simulink model "mCSControls_DG"  (R2012b)
settings: Solver=FixedStepDiscrete  StartTime=0.0  StopTime=10.0  RelTol=1e-3
values from neighbouring files (symbols this model uses):
  CDF2FThreshold = 45    [ControlCal_DG.m]
  CDF2TempThreshold = 20    [ControlCal_DG.m]
  delay = 5    [ControlCal_DG.m]
  DFThresh = 33    [ControlCal_DG.m]
  H = [90 90 90 90]    [ControlCal_DG.m]
  HeatTempThresh1 = 40    [ControlCal_DG.m]
  HeatTempThresh2 = 30    [ControlCal_DG.m]
  HeatTempThresh3 = 20    [ControlCal_DG.m]
  HStabilizationTime = 2*60    (= 120)    [ControlCal_DG.m]
  I_FAN = -1    [ControlCal_DG.m]
  I_VALVE = -1    [ControlCal_DG.m]
  initialSet = [1 1 1]    [ControlCal_DG.m]
  PBFTempThreshold = 30    [ControlCal_DG.m]
  PowerModeSwitchDelay = 30    [ControlCal_DG.m]
  SVocThresh = 550    [ControlCal_DG.m]
  T = [0 4 7 10]    [ControlCal_DG.m]
  Ts = 0.5    [ControlCal_DG.m]
  TSTempSetPoint = -2    [ControlCal_DG.m]
  TV1FThresh = 45    [ControlCal_DG.m]
  TV2FThresh = 60    [ControlCal_DG.m]
  VbatThresh = 22    [ControlCal_DG.m]
  VocDecRate = 0.5    [ControlCal_DG.m]
  VocIncrement = 5    [ControlCal_DG.m]
libraries: c2833xlib x29, simulink x23, c280xlib x11, idelinklib_tgtpref x1
(part 2 of 4)

== system mCSControls_DG/Inputs/EEPROM/EEPROMRead/AddressWrite ==
  Trigger : TriggerPort  PortDimensions=1
  Data Type Conversion : DataTypeConversion  OutDataTypeStr=uint8  RndMeth=Simplest
  I2C Transmit : c280xlib/I2C Transmit  addrFormat=7-Bit addressing  saSource=Specify via dialog  SAR=80  bitCount=8  STP=on  RM=off  STR=off
  WordAddress : Constant  Value=0  SampleTime=-1
  wires:
  WordAddress/1 -> Data Type Conversion/1
  Data Type Conversion/1 -> I2C Transmit/1

== system mCSControls_DG/Inputs/EEPROM/EEPROMRead/Receive ==
  Trigger : TriggerPort  TriggerType=falling  PortDimensions=1
  I2C Receive : c280xlib/I2C Receive  addrFormat=7-Bit addressing  saSource=Specify via dialog  SAR=80  bitCount=8  dataLength=3  initValue=initialSet  NACK=off  STP=on  STR=off  sampleTime=-1  dataType=uint8
  RD : Outport
  wires:
  I2C Receive/1 -> RD/1

== matlab function mCSControls_DG/Inputs/HMI/Data Detection ==
  data: u input; B output; M1 output; P1 output; Bp input; M1p input; P1p input
function [B,M1,P1] = fcn(u,Bp,M1p,P1p)
%#codegen

% When data length is 5 and format is [250 B M1 P 250]

n=5;
B=Bp;
M1=M1p;
P1=P1p;
for i=0:n-1
    if (u(i+1)==250 && u(mod(i+4,5)+1)==250)
        B  = u(mod(i+1,5)+1);
        M1 = u(mod(i+2,5)+1);
        P1 = u(mod(i+3,5)+1);
    end
end

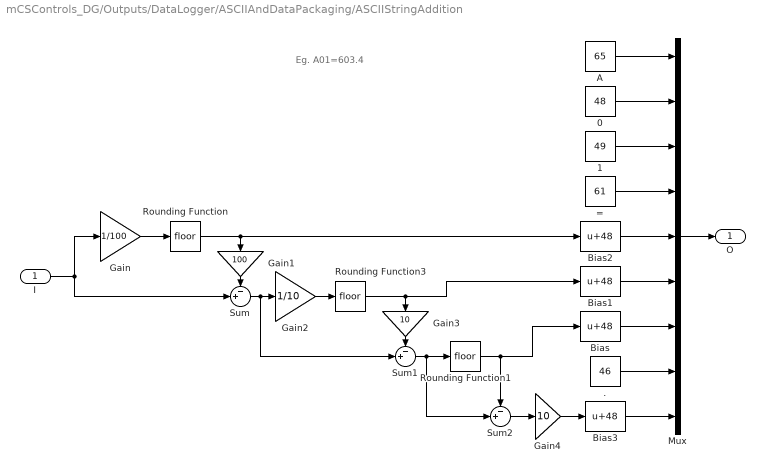
== system mCSControls_DG/Outputs/DataLogger/ASCIIAndDataPackaging/ASCIIStringAddition ==
  note: Eg. A01=603.4
  I : Inport
  . : Constant  Value=46
  0 : Constant  Value=48
  1 : Constant  Value=49
  = : Constant  Value=61
  A : Constant  Value=65
  Bias{,1..3} (4 alike) : Bias  Bias=48
  Gain : Gain  Gain=1/100
  Gain1 : Gain  Gain=100
  Gain2 : Gain  Gain=1/10
  Gain3 : Gain  Gain=10
  Gain4 : Gain  Gain=10
  Mux : Mux  Inputs=9
  Rounding Function : Rounding
  Rounding Function1 : Rounding
  Rounding Function3 : Rounding
  Sum : Sum  Inputs=-+|
  Sum1 : Sum  Inputs=-+|
  Sum2 : Sum  Inputs=-+|
  O : Outport
  wires:
  Gain3/1 -> Sum1/1
  Rounding Function3/1 -> Gain3/1, Bias1/1
  Gain2/1 -> Rounding Function3/1
  Sum/1 -> Gain2/1, Sum1/2
  Rounding Function/1 -> Gain1/1, Bias2/1
  Gain1/1 -> Sum/1
  I/1 -> Gain/1, Sum/2
  Gain/1 -> Rounding Function/1
  Mux/1 -> O/1
  A/1 -> Mux/1
  0/1 -> Mux/2
  1/1 -> Mux/3
  =/1 -> Mux/4
  Bias2/1 -> Mux/5
  Bias1/1 -> Mux/6
  Bias/1 -> Mux/7
  ./1 -> Mux/8
  Bias3/1 -> Mux/9
  Sum1/1 -> Sum2/2, Rounding Function1/1
  Rounding Function1/1 -> Bias/1, Sum2/1
  Sum2/1 -> Gain4/1
  Gain4/1 -> Bias3/1

== system mCSControls_DG/Outputs/DataLogger/ASCIIAndDataPackaging/ASCIIStringAddition1 ==
  note: Eg. &A02=26.4
  I : Inport
  & : Constant  Value=38
  . : Constant  Value=46
  0 : Constant  Value=48
  2 : Constant  Value=50
  = : Constant  Value=61
  A : Constant  Value=65
  Bias : Bias  Bias=48
  Bias1 : Bias  Bias=48
  Bias3 : Bias  Bias=48
  Gain2 : Gain  Gain=1/10
  Gain3 : Gain  Gain=10
  Gain4 : Gain  Gain=10
  Mux : Mux  Inputs=9
  Rounding Function1 : Rounding
  Rounding Function3 : Rounding
  Sum1 : Sum  Inputs=-+|
  Sum2 : Sum  Inputs=-+|
  O : Outport
  wires:
  Gain4/1 -> Bias3/1
  Sum2/1 -> Gain4/1
  Rounding Function1/1 -> Sum2/1, Bias/1
  Sum1/1 -> Rounding Function1/1, Sum2/2
  Mux/1 -> O/1
  I/1 -> Sum1/2, Gain2/1
  Gain2/1 -> Rounding Function3/1
  Rounding Function3/1 -> Bias1/1, Gain3/1
  Gain3/1 -> Sum1/1
  Bias3/1 -> Mux/9
  ./1 -> Mux/8
  Bias/1 -> Mux/7
  Bias1/1 -> Mux/6
  0/1 -> Mux/3
  =/1 -> Mux/5
  2/1 -> Mux/4
  A/1 -> Mux/2
  &/1 -> Mux/1

== system mCSControls_DG/Outputs/DataLogger/ASCIIAndDataPackaging/ASCIIStringAddition10 ==
  note: Eg. &A11=65.2
  I : Inport
  & : Constant  Value=38
  . : Constant  Value=46
  1 : Constant  Value=49
  = : Constant  Value=61
  A : Constant  Value=65
  Bias : Bias  Bias=48
  Bias1 : Bias  Bias=48
  Bias3 : Bias  Bias=48
  Gain2 : Gain  Gain=1/10
  Gain3 : Gain  Gain=10
  Gain4 : Gain  Gain=10
  Mux : Mux  Inputs=9
  Rounding Function1 : Rounding
  Rounding Function3 : Rounding
  Sum1 : Sum  Inputs=-+|
  Sum2 : Sum  Inputs=-+|
  one : Constant  Value=49
  O : Outport
  wires:
  Gain4/1 -> Bias3/1
  Sum2/1 -> Gain4/1
  Rounding Function1/1 -> Sum2/1, Bias/1
  Sum1/1 -> Rounding Function1/1, Sum2/2
  Mux/1 -> O/1
  I/1 -> Sum1/2, Gain2/1
  Gain2/1 -> Rounding Function3/1
  Rounding Function3/1 -> Bias1/1, Gain3/1
  Gain3/1 -> Sum1/1
  Bias3/1 -> Mux/9
  ./1 -> Mux/8
  Bias/1 -> Mux/7
  Bias1/1 -> Mux/6
  1/1 -> Mux/3
  =/1 -> Mux/5
  one/1 -> Mux/4
  A/1 -> Mux/2
  &/1 -> Mux/1

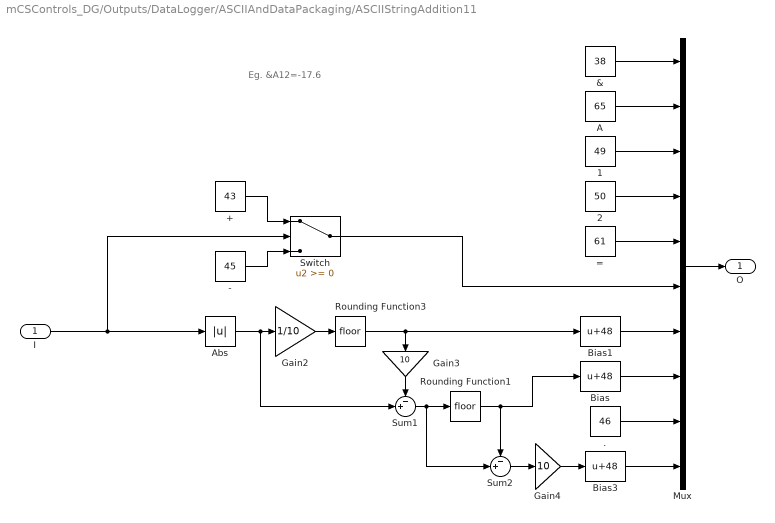
== system mCSControls_DG/Outputs/DataLogger/ASCIIAndDataPackaging/ASCIIStringAddition11 ==
  note: Eg. &A12=-17.6
  I : Inport
  & : Constant  Value=38
  + : Constant  Value=43
  - : Constant  Value=45
  . : Constant  Value=46
  1 : Constant  Value=49
  2 : Constant  Value=50
  = : Constant  Value=61
  A : Constant  Value=65
  Abs : Abs
  Bias : Bias  Bias=48
  Bias1 : Bias  Bias=48
  Bias3 : Bias  Bias=48
  Gain2 : Gain  Gain=1/10
  Gain3 : Gain  Gain=10
  Gain4 : Gain  Gain=10
  Mux : Mux  Inputs=10
  Rounding Function1 : Rounding
  Rounding Function3 : Rounding
  Sum1 : Sum  Inputs=-+|
  Sum2 : Sum  Inputs=-+|
  Switch : Switch
  O : Outport
  wires:
  Gain4/1 -> Bias3/1
  Sum2/1 -> Gain4/1
  Rounding Function1/1 -> Sum2/1, Bias/1
  Sum1/1 -> Rounding Function1/1, Sum2/2
  Mux/1 -> O/1
  Gain2/1 -> Rounding Function3/1
  Rounding Function3/1 -> Gain3/1, Bias1/1
  Gain3/1 -> Sum1/1
  Abs/1 -> Sum1/2, Gain2/1
  -/1 -> Switch/3
  +/1 -> Switch/1
  I/1 -> Switch/2, Abs/1
  &/1 -> Mux/1
  A/1 -> Mux/2
  1/1 -> Mux/3
  2/1 -> Mux/4
  =/1 -> Mux/5
  Switch/1 -> Mux/6
  Bias3/1 -> Mux/10
  Bias1/1 -> Mux/7
  Bias/1 -> Mux/8
  ./1 -> Mux/9

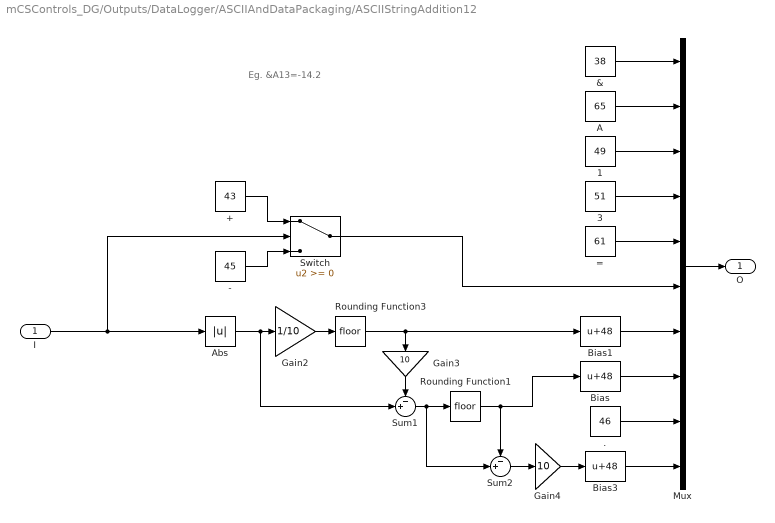
== system mCSControls_DG/Outputs/DataLogger/ASCIIAndDataPackaging/ASCIIStringAddition12 ==
  note: Eg. &A13=-14.2
  I : Inport
  & : Constant  Value=38
  + : Constant  Value=43
  - : Constant  Value=45
  . : Constant  Value=46
  1 : Constant  Value=49
  3 : Constant  Value=51
  = : Constant  Value=61
  A : Constant  Value=65
  Abs : Abs
  Bias : Bias  Bias=48
  Bias1 : Bias  Bias=48
  Bias3 : Bias  Bias=48
  Gain2 : Gain  Gain=1/10
  Gain3 : Gain  Gain=10
  Gain4 : Gain  Gain=10
  Mux : Mux  Inputs=10
  Rounding Function1 : Rounding
  Rounding Function3 : Rounding
  Sum1 : Sum  Inputs=-+|
  Sum2 : Sum  Inputs=-+|
  Switch : Switch
  O : Outport
  wires:
  ./1 -> Mux/9
  Bias/1 -> Mux/8
  Bias1/1 -> Mux/7
  Bias3/1 -> Mux/10
  Switch/1 -> Mux/6
  =/1 -> Mux/5
  3/1 -> Mux/4
  1/1 -> Mux/3
  A/1 -> Mux/2
  &/1 -> Mux/1
  I/1 -> Abs/1, Switch/2
  +/1 -> Switch/1
  -/1 -> Switch/3
  Abs/1 -> Gain2/1, Sum1/2
  Gain3/1 -> Sum1/1
  Rounding Function3/1 -> Bias1/1, Gain3/1
  Gain2/1 -> Rounding Function3/1
  Mux/1 -> O/1
  Sum1/1 -> Sum2/2, Rounding Function1/1
  Rounding Function1/1 -> Bias/1, Sum2/1
  Sum2/1 -> Gain4/1
  Gain4/1 -> Bias3/1

== system mCSControls_DG/Outputs/DataLogger/ASCIIAndDataPackaging/ASCIIStringAddition13 ==
  note: Eg. &A14=86.9
  I : Inport
  & : Constant  Value=38
  . : Constant  Value=46
  1 : Constant  Value=49
  4 : Constant  Value=52
  = : Constant  Value=61
  A : Constant  Value=65
  Bias : Bias  Bias=48
  Bias1 : Bias  Bias=48
  Bias3 : Bias  Bias=48
  Gain2 : Gain  Gain=1/10
  Gain3 : Gain  Gain=10
  Gain4 : Gain  Gain=10
  Mux : Mux  Inputs=9
  Rounding Function1 : Rounding
  Rounding Function3 : Rounding
  Sum1 : Sum  Inputs=-+|
  Sum2 : Sum  Inputs=-+|
  O : Outport
  wires:
  &/1 -> Mux/1
  A/1 -> Mux/2
  4/1 -> Mux/4
  =/1 -> Mux/5
  1/1 -> Mux/3
  Bias1/1 -> Mux/6
  Bias/1 -> Mux/7
  ./1 -> Mux/8
  Bias3/1 -> Mux/9
  Gain3/1 -> Sum1/1
  Rounding Function3/1 -> Gain3/1, Bias1/1
  Gain2/1 -> Rounding Function3/1
  I/1 -> Gain2/1, Sum1/2
  Mux/1 -> O/1
  Sum1/1 -> Sum2/2, Rounding Function1/1
  Rounding Function1/1 -> Bias/1, Sum2/1
  Sum2/1 -> Gain4/1
  Gain4/1 -> Bias3/1

== system mCSControls_DG/Outputs/DataLogger/ASCIIAndDataPackaging/ASCIIStringAddition14 ==
  note: Eg. &A15=51.2
  I : Inport
  & : Constant  Value=38
  . : Constant  Value=46
  1 : Constant  Value=49
  5 : Constant  Value=53
  = : Constant  Value=61
  A : Constant  Value=65
  Bias : Bias  Bias=48
  Bias1 : Bias  Bias=48
  Bias3 : Bias  Bias=48
  Gain2 : Gain  Gain=1/10
  Gain3 : Gain  Gain=10
  Gain4 : Gain  Gain=10
  Mux : Mux  Inputs=9
  Rounding Function1 : Rounding
  Rounding Function3 : Rounding
  Sum1 : Sum  Inputs=-+|
  Sum2 : Sum  Inputs=-+|
  O : Outport
  wires:
  Gain4/1 -> Bias3/1
  Sum2/1 -> Gain4/1
  Rounding Function1/1 -> Sum2/1, Bias/1
  Sum1/1 -> Rounding Function1/1, Sum2/2
  Mux/1 -> O/1
  I/1 -> Sum1/2, Gain2/1
  Gain2/1 -> Rounding Function3/1
  Rounding Function3/1 -> Bias1/1, Gain3/1
  Gain3/1 -> Sum1/1
  Bias3/1 -> Mux/9
  ./1 -> Mux/8
  Bias/1 -> Mux/7
  Bias1/1 -> Mux/6
  1/1 -> Mux/3
  =/1 -> Mux/5
  5/1 -> Mux/4
  A/1 -> Mux/2
  &/1 -> Mux/1

== system mCSControls_DG/Outputs/DataLogger/ASCIIAndDataPackaging/ASCIIStringAddition15 ==
  note: Eg. &A38=159
  I : Inport
  & : Constant  Value=38
  3 : Constant  Value=51
  8 : Constant  Value=56
  = : Constant  Value=61
  A : Constant  Value=65
  Bias : Bias  Bias=48
  Bias1 : Bias  Bias=48
  Bias3 : Bias  Bias=48
  Gain1 : Gain  Gain=1/10
  Gain2 : Gain  Gain=1/100
  Gain3 : Gain  Gain=100
  Gain4 : Gain  Gain=10
  Mux : Mux  Inputs=8
  Rounding Function1 : Rounding
  Rounding Function2 : Rounding
  Rounding Function3 : Rounding
  Sum1 : Sum  Inputs=-+|
  Sum2 : Sum  Inputs=-+|
  O : Outport
  wires:
  &/1 -> Mux/1
  A/1 -> Mux/2
  8/1 -> Mux/4
  =/1 -> Mux/5
  3/1 -> Mux/3
  Bias1/1 -> Mux/6
  Bias/1 -> Mux/7
  Bias3/1 -> Mux/8
  Gain3/1 -> Sum1/1
  Rounding Function3/1 -> Bias1/1, Gain3/1
  Gain2/1 -> Rounding Function3/1
  I/1 -> Gain2/1, Sum1/2
  Mux/1 -> O/1
  Sum1/1 -> Sum2/2, Gain1/1
  Rounding Function1/1 -> Bias/1, Gain4/1
  Sum2/1 -> Rounding Function2/1
  Gain1/1 -> Rounding Function1/1
  Gain4/1 -> Sum2/1
  Rounding Function2/1 -> Bias3/1

== system mCSControls_DG/Outputs/DataLogger/ASCIIAndDataPackaging/ASCIIStringAddition16 ==
  note: Eg. &A17=3.4
  I : Inport
  & : Constant  Value=38
  . : Constant  Value=46
  1 : Constant  Value=49
  7 : Constant  Value=55
  = : Constant  Value=61
  A : Constant  Value=65
  Bias : Bias  Bias=48
  Bias3 : Bias  Bias=48
  Gain4 : Gain  Gain=10
  Mux : Mux  Inputs=8
  Rounding Function1 : Rounding
  Sum2 : Sum  Inputs=-+|
  O : Outport
  wires:
  Gain4/1 -> Bias3/1
  Sum2/1 -> Gain4/1
  Rounding Function1/1 -> Sum2/1, Bias/1
  I/1 -> Rounding Function1/1, Sum2/2
  Mux/1 -> O/1
  &/1 -> Mux/1
  A/1 -> Mux/2
  1/1 -> Mux/3
  7/1 -> Mux/4
  =/1 -> Mux/5
  Bias/1 -> Mux/6
  ./1 -> Mux/7
  Bias3/1 -> Mux/8

== system mCSControls_DG/Outputs/DataLogger/ASCIIAndDataPackaging/ASCIIStringAddition17 ==
  note: Eg. &A18=0
  I : Inport
  & : Constant  Value=38
  1 : Constant  Value=49
  8 : Constant  Value=56
  = : Constant  Value=61
  A : Constant  Value=65
  Bias1 : Bias  Bias=48
  Mux : Mux  Inputs=6
  O : Outport
  wires:
  I/1 -> Bias1/1
  Mux/1 -> O/1
  Bias1/1 -> Mux/6
  1/1 -> Mux/3
  =/1 -> Mux/5
  8/1 -> Mux/4
  A/1 -> Mux/2
  &/1 -> Mux/1

== system mCSControls_DG/Outputs/DataLogger/ASCIIAndDataPackaging/ASCIIStringAddition18 ==
  note: Eg. &A19=0
  I : Inport
  & : Constant  Value=38
  1 : Constant  Value=49
  9 : Constant  Value=57
  = : Constant  Value=61
  A : Constant  Value=65
  Bias1 : Bias  Bias=48
  Mux : Mux  Inputs=6
  O : Outport
  wires:
  &/1 -> Mux/1
  A/1 -> Mux/2
  9/1 -> Mux/4
  =/1 -> Mux/5
  1/1 -> Mux/3
  Bias1/1 -> Mux/6
  Mux/1 -> O/1
  I/1 -> Bias1/1

== system mCSControls_DG/Outputs/DataLogger/ASCIIAndDataPackaging/ASCIIStringAddition19 ==
  note: Eg. &A20=0
  I : Inport
  & : Constant  Value=38
  0 : Constant  Value=48
  2 : Constant  Value=50
  = : Constant  Value=61
  A : Constant  Value=65
  Bias1 : Bias  Bias=48
  Mux : Mux  Inputs=6
  O : Outport
  wires:
  I/1 -> Bias1/1
  Mux/1 -> O/1
  Bias1/1 -> Mux/6
  2/1 -> Mux/3
  =/1 -> Mux/5
  0/1 -> Mux/4
  A/1 -> Mux/2
  &/1 -> Mux/1

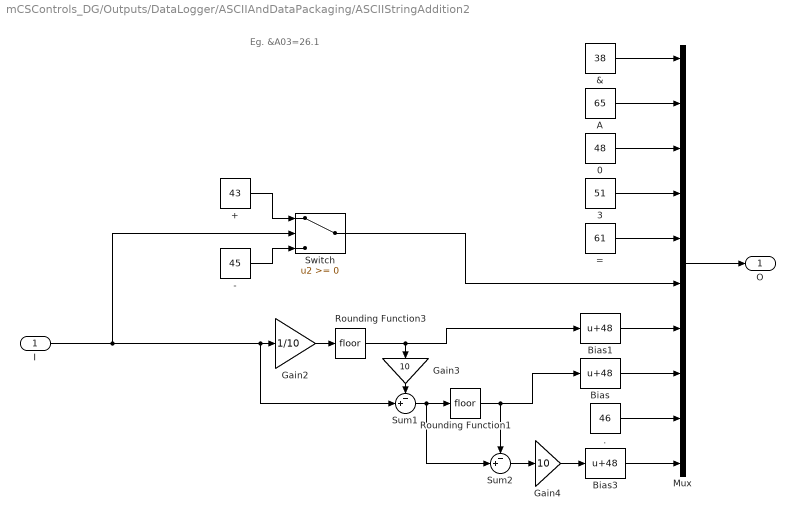
== system mCSControls_DG/Outputs/DataLogger/ASCIIAndDataPackaging/ASCIIStringAddition2 ==
  note: Eg. &A03=26.1
  I : Inport
  & : Constant  Value=38
  + : Constant  Value=43
  - : Constant  Value=45
  . : Constant  Value=46
  0 : Constant  Value=48
  3 : Constant  Value=51
  = : Constant  Value=61
  A : Constant  Value=65
  Bias : Bias  Bias=48
  Bias1 : Bias  Bias=48
  Bias3 : Bias  Bias=48
  Gain2 : Gain  Gain=1/10
  Gain3 : Gain  Gain=10
  Gain4 : Gain  Gain=10
  Mux : Mux  Inputs=10
  Rounding Function1 : Rounding
  Rounding Function3 : Rounding
  Sum1 : Sum  Inputs=-+|
  Sum2 : Sum  Inputs=-+|
  Switch : Switch
  O : Outport
  wires:
  &/1 -> Mux/1
  A/1 -> Mux/2
  3/1 -> Mux/4
  =/1 -> Mux/5
  0/1 -> Mux/3
  Gain3/1 -> Sum1/1
  Rounding Function3/1 -> Gain3/1, Bias1/1
  Gain2/1 -> Rounding Function3/1
  Mux/1 -> O/1
  Sum1/1 -> Sum2/2, Rounding Function1/1
  Rounding Function1/1 -> Bias/1, Sum2/1
  Sum2/1 -> Gain4/1
  Gain4/1 -> Bias3/1
  Bias3/1 -> Mux/10
  ./1 -> Mux/9
  Bias/1 -> Mux/8
  Bias1/1 -> Mux/7
  Switch/1 -> Mux/6
  I/1 -> Switch/2, Gain2/1, Sum1/2
  +/1 -> Switch/1
  -/1 -> Switch/3

== system mCSControls_DG/Outputs/DataLogger/ASCIIAndDataPackaging/ASCIIStringAddition20 ==
  note: Eg. &A21=0
  I : Inport
  & : Constant  Value=38
  1 : Constant  Value=49
  2 : Constant  Value=50
  = : Constant  Value=61
  A : Constant  Value=65
  Bias1 : Bias  Bias=48
  Mux : Mux  Inputs=6
  O : Outport
  wires:
  &/1 -> Mux/1
  A/1 -> Mux/2
  1/1 -> Mux/4
  =/1 -> Mux/5
  2/1 -> Mux/3
  Bias1/1 -> Mux/6
  Mux/1 -> O/1
  I/1 -> Bias1/1

== system mCSControls_DG/Outputs/DataLogger/ASCIIAndDataPackaging/ASCIIStringAddition21 ==
  note: Eg. &A22=0
  I : Inport
  & : Constant  Value=38
  2 : Constant  Value=50
  = : Constant  Value=61
  A : Constant  Value=65
  Bias1 : Bias  Bias=48
  Mux : Mux  Inputs=6
  two : Constant  Value=50
  O : Outport
  wires:
  I/1 -> Bias1/1
  Mux/1 -> O/1
  Bias1/1 -> Mux/6
  2/1 -> Mux/3
  =/1 -> Mux/5
  two/1 -> Mux/4
  A/1 -> Mux/2
  &/1 -> Mux/1

== system mCSControls_DG/Outputs/DataLogger/ASCIIAndDataPackaging/ASCIIStringAddition22 ==
  note: Eg. &A23=0
  I : Inport
  & : Constant  Value=38
  2 : Constant  Value=50
  3 : Constant  Value=51
  = : Constant  Value=61
  A : Constant  Value=65
  Bias1 : Bias  Bias=48
  Mux : Mux  Inputs=6
  O : Outport
  wires:
  &/1 -> Mux/1
  A/1 -> Mux/2
  3/1 -> Mux/4
  =/1 -> Mux/5
  2/1 -> Mux/3
  Bias1/1 -> Mux/6
  Mux/1 -> O/1
  I/1 -> Bias1/1

== system mCSControls_DG/Outputs/DataLogger/ASCIIAndDataPackaging/ASCIIStringAddition23 ==
  note: Eg. &A24=0
  I : Inport
  & : Constant  Value=38
  2 : Constant  Value=50
  4 : Constant  Value=52
  = : Constant  Value=61
  A : Constant  Value=65
  Bias1 : Bias  Bias=48
  Mux : Mux  Inputs=6
  O : Outport
  wires:
  I/1 -> Bias1/1
  Mux/1 -> O/1
  Bias1/1 -> Mux/6
  2/1 -> Mux/3
  =/1 -> Mux/5
  4/1 -> Mux/4
  A/1 -> Mux/2
  &/1 -> Mux/1

== system mCSControls_DG/Outputs/DataLogger/ASCIIAndDataPackaging/ASCIIStringAddition24 ==
  note: Eg. &A25=0
  I : Inport
  & : Constant  Value=38
  2 : Constant  Value=50
  5 : Constant  Value=53
  = : Constant  Value=61
  A : Constant  Value=65
  Bias1 : Bias  Bias=48
  Mux : Mux  Inputs=6
  O : Outport
  wires:
  &/1 -> Mux/1
  A/1 -> Mux/2
  5/1 -> Mux/4
  =/1 -> Mux/5
  2/1 -> Mux/3
  Bias1/1 -> Mux/6
  Mux/1 -> O/1
  I/1 -> Bias1/1

== system mCSControls_DG/Outputs/DataLogger/ASCIIAndDataPackaging/ASCIIStringAddition25 ==
  note: Eg. &A26=0
  I : Inport
  & : Constant  Value=38
  2 : Constant  Value=50
  6 : Constant  Value=54
  = : Constant  Value=61
  A : Constant  Value=65
  Bias1 : Bias  Bias=48
  Mux : Mux  Inputs=6
  O : Outport
  wires:
  I/1 -> Bias1/1
  Mux/1 -> O/1
  Bias1/1 -> Mux/6
  2/1 -> Mux/3
  =/1 -> Mux/5
  6/1 -> Mux/4
  A/1 -> Mux/2
  &/1 -> Mux/1

== system mCSControls_DG/Outputs/DataLogger/ASCIIAndDataPackaging/ASCIIStringAddition26 ==
  note: Eg. &A27=0
  I : Inport
  & : Constant  Value=38
  2 : Constant  Value=50
  7 : Constant  Value=55
  = : Constant  Value=61
  A : Constant  Value=65
  Bias1 : Bias  Bias=48
  Mux : Mux  Inputs=6
  O : Outport
  wires:
  &/1 -> Mux/1
  A/1 -> Mux/2
  7/1 -> Mux/4
  =/1 -> Mux/5
  2/1 -> Mux/3
  Bias1/1 -> Mux/6
  Mux/1 -> O/1
  I/1 -> Bias1/1

== system mCSControls_DG/Outputs/DataLogger/ASCIIAndDataPackaging/ASCIIStringAddition27 ==
  note: Eg. &A28=0
  I : Inport
  & : Constant  Value=38
  2 : Constant  Value=50
  8 : Constant  Value=56
  = : Constant  Value=61
  A : Constant  Value=65
  Bias1 : Bias  Bias=48
  Mux : Mux  Inputs=6
  O : Outport
  wires:
  I/1 -> Bias1/1
  Mux/1 -> O/1
  Bias1/1 -> Mux/6
  2/1 -> Mux/3
  =/1 -> Mux/5
  8/1 -> Mux/4
  A/1 -> Mux/2
  &/1 -> Mux/1

== system mCSControls_DG/Outputs/DataLogger/ASCIIAndDataPackaging/ASCIIStringAddition28 ==
  note: Eg. &A29=0
  I : Inport
  & : Constant  Value=38
  2 : Constant  Value=50
  9 : Constant  Value=57
  = : Constant  Value=61
  A : Constant  Value=65
  Bias1 : Bias  Bias=48
  Mux : Mux  Inputs=6
  O : Outport
  wires:
  &/1 -> Mux/1
  A/1 -> Mux/2
  9/1 -> Mux/4
  =/1 -> Mux/5
  2/1 -> Mux/3
  Bias1/1 -> Mux/6
  Mux/1 -> O/1
  I/1 -> Bias1/1

== system mCSControls_DG/Outputs/DataLogger/ASCIIAndDataPackaging/ASCIIStringAddition29 ==
  note: Eg. &A30=0
  I : Inport
  & : Constant  Value=38
  0 : Constant  Value=48
  3 : Constant  Value=51
  = : Constant  Value=61
  A : Constant  Value=65
  Bias1 : Bias  Bias=48
  Mux : Mux  Inputs=6
  O : Outport
  wires:
  I/1 -> Bias1/1
  Mux/1 -> O/1
  Bias1/1 -> Mux/6
  3/1 -> Mux/3
  =/1 -> Mux/5
  0/1 -> Mux/4
  A/1 -> Mux/2
  &/1 -> Mux/1

== system mCSControls_DG/Outputs/DataLogger/ASCIIAndDataPackaging/ASCIIStringAddition3 ==
  note: Eg. &A04=60.1
  I : Inport
  & : Constant  Value=38
  + : Constant  Value=43
  - : Constant  Value=45
  . : Constant  Value=46
  0 : Constant  Value=48
  4 : Constant  Value=52
  = : Constant  Value=61
  A : Constant  Value=65
  Bias : Bias  Bias=48
  Bias1 : Bias  Bias=48
  Bias3 : Bias  Bias=48
  Gain2 : Gain  Gain=1/10
  Gain3 : Gain  Gain=10
  Gain4 : Gain  Gain=10
  Mux : Mux  Inputs=10
  Rounding Function1 : Rounding
  Rounding Function3 : Rounding
  Sum1 : Sum  Inputs=-+|
  Sum2 : Sum  Inputs=-+|
  Switch : Switch
  O : Outport
  wires:
  Gain4/1 -> Bias3/1
  Sum2/1 -> Gain4/1
  Rounding Function1/1 -> Sum2/1, Bias/1
  Sum1/1 -> Rounding Function1/1, Sum2/2
  Mux/1 -> O/1
  Gain2/1 -> Rounding Function3/1
  Rounding Function3/1 -> Bias1/1, Gain3/1
  Gain3/1 -> Sum1/1
  0/1 -> Mux/3
  =/1 -> Mux/5
  4/1 -> Mux/4
  A/1 -> Mux/2
  &/1 -> Mux/1
  Bias1/1 -> Mux/7
  Bias/1 -> Mux/8
  ./1 -> Mux/9
  Bias3/1 -> Mux/10
  Switch/1 -> Mux/6
  I/1 -> Switch/2, Sum1/2, Gain2/1
  +/1 -> Switch/1
  -/1 -> Switch/3

== system mCSControls_DG/Outputs/DataLogger/ASCIIAndDataPackaging/ASCIIStringAddition30 ==
  note: Eg. &A31=0
  I : Inport
  & : Constant  Value=38
  1 : Constant  Value=49
  3 : Constant  Value=51
  = : Constant  Value=61
  A : Constant  Value=65
  Bias1 : Bias  Bias=48
  Mux : Mux  Inputs=6
  O : Outport
  wires:
  &/1 -> Mux/1
  A/1 -> Mux/2
  1/1 -> Mux/4
  =/1 -> Mux/5
  3/1 -> Mux/3
  Bias1/1 -> Mux/6
  Mux/1 -> O/1
  I/1 -> Bias1/1

== system mCSControls_DG/Outputs/DataLogger/ASCIIAndDataPackaging/ASCIIStringAddition31 ==
  note: Eg. &A32=0
  I : Inport
  & : Constant  Value=38
  2 : Constant  Value=50
  3 : Constant  Value=51
  = : Constant  Value=61
  A : Constant  Value=65
  Bias1 : Bias  Bias=48
  Mux : Mux  Inputs=6
  O : Outport
  wires:
  I/1 -> Bias1/1
  Mux/1 -> O/1
  Bias1/1 -> Mux/6
  3/1 -> Mux/3
  =/1 -> Mux/5
  2/1 -> Mux/4
  A/1 -> Mux/2
  &/1 -> Mux/1

== system mCSControls_DG/Outputs/DataLogger/ASCIIAndDataPackaging/ASCIIStringAddition32 ==
  note: Eg. &A33=0
  I : Inport
  & : Constant  Value=38
  3 : Constant  Value=51
  = : Constant  Value=61
  A : Constant  Value=65
  Bias1 : Bias  Bias=48
  Mux : Mux  Inputs=6
  three : Constant  Value=51
  O : Outport
  wires:
  &/1 -> Mux/1
  A/1 -> Mux/2
  three/1 -> Mux/4
  =/1 -> Mux/5
  3/1 -> Mux/3
  Bias1/1 -> Mux/6
  Mux/1 -> O/1
  I/1 -> Bias1/1

== system mCSControls_DG/Outputs/DataLogger/ASCIIAndDataPackaging/ASCIIStringAddition33 ==
  note: Eg. &A34=0
  I : Inport
  & : Constant  Value=38
  3 : Constant  Value=51
  4 : Constant  Value=52
  = : Constant  Value=61
  A : Constant  Value=65
  Bias1 : Bias  Bias=48
  Mux : Mux  Inputs=6
  O : Outport
  wires:
  I/1 -> Bias1/1
  Mux/1 -> O/1
  Bias1/1 -> Mux/6
  3/1 -> Mux/3
  =/1 -> Mux/5
  4/1 -> Mux/4
  A/1 -> Mux/2
  &/1 -> Mux/1

== system mCSControls_DG/Outputs/DataLogger/ASCIIAndDataPackaging/ASCIIStringAddition34 ==
  note: Eg. &A35=0
  I : Inport
  & : Constant  Value=38
  3 : Constant  Value=51
  5 : Constant  Value=53
  = : Constant  Value=61
  A : Constant  Value=65
  Bias1 : Bias  Bias=48
  Mux : Mux  Inputs=6
  O : Outport
  wires:
  &/1 -> Mux/1
  A/1 -> Mux/2
  5/1 -> Mux/4
  =/1 -> Mux/5
  3/1 -> Mux/3
  Bias1/1 -> Mux/6
  Mux/1 -> O/1
  I/1 -> Bias1/1

== system mCSControls_DG/Outputs/DataLogger/ASCIIAndDataPackaging/ASCIIStringAddition35 ==
  note: Eg. &A36=0
  I : Inport
  & : Constant  Value=38
  3 : Constant  Value=51
  6 : Constant  Value=54
  = : Constant  Value=61
  A : Constant  Value=65
  Bias1 : Bias  Bias=48
  Mux : Mux  Inputs=6
  O : Outport
  wires:
  I/1 -> Bias1/1
  Mux/1 -> O/1
  Bias1/1 -> Mux/6
  3/1 -> Mux/3
  =/1 -> Mux/5
  6/1 -> Mux/4
  A/1 -> Mux/2
  &/1 -> Mux/1

== system mCSControls_DG/Outputs/DataLogger/ASCIIAndDataPackaging/ASCIIStringAddition36 ==
  note: Eg. &A37=0
  I : Inport
  & : Constant  Value=38
  3 : Constant  Value=51
  7 : Constant  Value=55
  = : Constant  Value=61
  A : Constant  Value=65
  Bias1 : Bias  Bias=48
  Mux : Mux  Inputs=6
  O : Outport
  wires:
  &/1 -> Mux/1
  A/1 -> Mux/2
  7/1 -> Mux/4
  =/1 -> Mux/5
  3/1 -> Mux/3
  Bias1/1 -> Mux/6
  Mux/1 -> O/1
  I/1 -> Bias1/1

== system mCSControls_DG/Outputs/DataLogger/ASCIIAndDataPackaging/ASCIIStringAddition37 ==
  note: Eg. &A16=7.1
  I : Inport
  & : Constant  Value=38
  . : Constant  Value=46
  1 : Constant  Value=49
  6 : Constant  Value=54
  = : Constant  Value=61
  A : Constant  Value=65
  Bias : Bias  Bias=48
  Bias3 : Bias  Bias=48
  Gain4 : Gain  Gain=10
  Mux : Mux  Inputs=8
  Rounding Function1 : Rounding
  Sum2 : Sum  Inputs=-+|
  O : Outport
  wires:
  Bias3/1 -> Mux/8
  ./1 -> Mux/7
  Bias/1 -> Mux/6
  =/1 -> Mux/5
  6/1 -> Mux/4
  1/1 -> Mux/3
  A/1 -> Mux/2
  &/1 -> Mux/1
  Mux/1 -> O/1
  I/1 -> Sum2/2, Rounding Function1/1
  Rounding Function1/1 -> Bias/1, Sum2/1
  Sum2/1 -> Gain4/1
  Gain4/1 -> Bias3/1

== system mCSControls_DG/Outputs/DataLogger/ASCIIAndDataPackaging/ASCIIStringAddition38 ==
  note: Eg. &A39=159
  I : Inport
  & : Constant  Value=38
  1 : Constant  Value=51
  9 : Constant  Value=57
  = : Constant  Value=61
  A : Constant  Value=65
  Bias : Bias  Bias=48
  Bias1 : Bias  Bias=48
  Bias3 : Bias  Bias=48
  Gain1 : Gain  Gain=1/10
  Gain2 : Gain  Gain=1/100
  Gain3 : Gain  Gain=100
  Gain4 : Gain  Gain=10
  Mux : Mux  Inputs=8
  Rounding Function1 : Rounding
  Rounding Function2 : Rounding
  Rounding Function3 : Rounding
  Sum1 : Sum  Inputs=-+|
  Sum2 : Sum  Inputs=-+|
  O : Outport
  wires:
  Rounding Function2/1 -> Bias3/1
  Gain4/1 -> Sum2/1
  Gain1/1 -> Rounding Function1/1
  Sum2/1 -> Rounding Function2/1
  Rounding Function1/1 -> Gain4/1, Bias/1
  Sum1/1 -> Gain1/1, Sum2/2
  Mux/1 -> O/1
  I/1 -> Sum1/2, Gain2/1
  Gain2/1 -> Rounding Function3/1
  Rounding Function3/1 -> Gain3/1, Bias1/1
  Gain3/1 -> Sum1/1
  Bias3/1 -> Mux/8
  Bias/1 -> Mux/7
  Bias1/1 -> Mux/6
  1/1 -> Mux/3
  =/1 -> Mux/5
  9/1 -> Mux/4
  A/1 -> Mux/2
  &/1 -> Mux/1

== system mCSControls_DG/Outputs/DataLogger/ASCIIAndDataPackaging/ASCIIStringAddition4 ==
  note: Eg. &A05=0
  I : Inport
  & : Constant  Value=38
  0 : Constant  Value=48
  5 : Constant  Value=53
  = : Constant  Value=61
  A : Constant  Value=65
  Bias1 : Bias  Bias=48
  Mux : Mux  Inputs=6
  O : Outport
  wires:
  &/1 -> Mux/1
  A/1 -> Mux/2
  5/1 -> Mux/4
  =/1 -> Mux/5
  0/1 -> Mux/3
  Bias1/1 -> Mux/6
  Mux/1 -> O/1
  I/1 -> Bias1/1

== system mCSControls_DG/Outputs/DataLogger/ASCIIAndDataPackaging/ASCIIStringAddition5 ==
  note: Eg. &A06=0
  I : Inport
  & : Constant  Value=38
  0 : Constant  Value=48
  6 : Constant  Value=54
  = : Constant  Value=61
  A : Constant  Value=65
  Bias1 : Bias  Bias=48
  Mux : Mux  Inputs=6
  O : Outport
  wires:
  I/1 -> Bias1/1
  Mux/1 -> O/1
  Bias1/1 -> Mux/6
  0/1 -> Mux/3
  =/1 -> Mux/5
  6/1 -> Mux/4
  A/1 -> Mux/2
  &/1 -> Mux/1

== system mCSControls_DG/Outputs/DataLogger/ASCIIAndDataPackaging/ASCIIStringAddition6 ==
  note: Eg. &A07=0
  I : Inport
  & : Constant  Value=38
  0 : Constant  Value=48
  7 : Constant  Value=55
  = : Constant  Value=61
  A : Constant  Value=65
  Bias1 : Bias  Bias=48
  Mux : Mux  Inputs=6
  O : Outport
  wires:
  &/1 -> Mux/1
  A/1 -> Mux/2
  7/1 -> Mux/4
  =/1 -> Mux/5
  0/1 -> Mux/3
  Bias1/1 -> Mux/6
  Mux/1 -> O/1
  I/1 -> Bias1/1

== system mCSControls_DG/Outputs/DataLogger/ASCIIAndDataPackaging/ASCIIStringAddition7 ==
  note: Eg. &A08=1
  I : Inport
  & : Constant  Value=38
  0 : Constant  Value=48
  8 : Constant  Value=56
  = : Constant  Value=61
  A : Constant  Value=65
  Bias1 : Bias  Bias=48
  Mux : Mux  Inputs=6
  O : Outport
  wires:
  I/1 -> Bias1/1
  Mux/1 -> O/1
  Bias1/1 -> Mux/6
  0/1 -> Mux/3
  =/1 -> Mux/5
  8/1 -> Mux/4
  A/1 -> Mux/2
  &/1 -> Mux/1

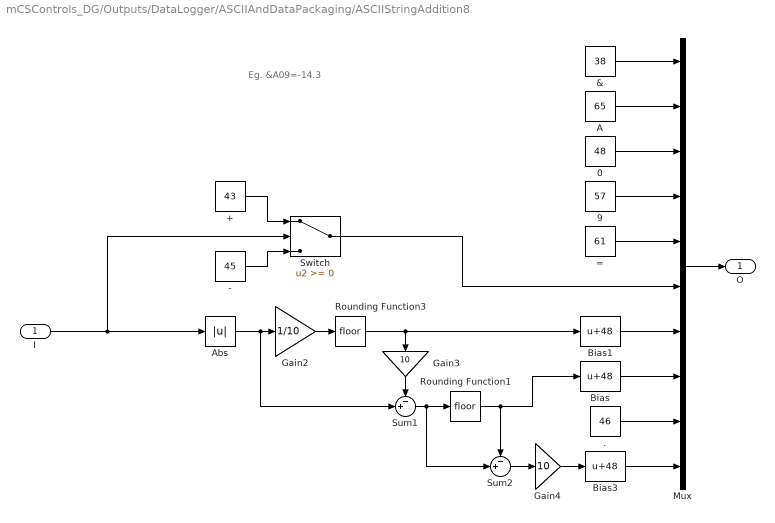
== system mCSControls_DG/Outputs/DataLogger/ASCIIAndDataPackaging/ASCIIStringAddition8 ==
  note: Eg. &A09=-14.3
  I : Inport
  & : Constant  Value=38
  + : Constant  Value=43
  - : Constant  Value=45
  . : Constant  Value=46
  0 : Constant  Value=48
  9 : Constant  Value=57
  = : Constant  Value=61
  A : Constant  Value=65
  Abs : Abs
  Bias : Bias  Bias=48
  Bias1 : Bias  Bias=48
  Bias3 : Bias  Bias=48
  Gain2 : Gain  Gain=1/10
  Gain3 : Gain  Gain=10
  Gain4 : Gain  Gain=10
  Mux : Mux  Inputs=10
  Rounding Function1 : Rounding
  Rounding Function3 : Rounding
  Sum1 : Sum  Inputs=-+|
  Sum2 : Sum  Inputs=-+|
  Switch : Switch
  O : Outport
  wires:
  Gain4/1 -> Bias3/1
  Sum2/1 -> Gain4/1
  Rounding Function1/1 -> Sum2/1, Bias/1
  Sum1/1 -> Rounding Function1/1, Sum2/2
  Mux/1 -> O/1
  Gain2/1 -> Rounding Function3/1
  Rounding Function3/1 -> Gain3/1, Bias1/1
  Gain3/1 -> Sum1/1
  Abs/1 -> Sum1/2, Gain2/1
  -/1 -> Switch/3
  +/1 -> Switch/1
  I/1 -> Switch/2, Abs/1
  &/1 -> Mux/1
  A/1 -> Mux/2
  0/1 -> Mux/3
  9/1 -> Mux/4
  =/1 -> Mux/5
  Switch/1 -> Mux/6
  Bias3/1 -> Mux/10
  Bias1/1 -> Mux/7
  Bias/1 -> Mux/8
  ./1 -> Mux/9

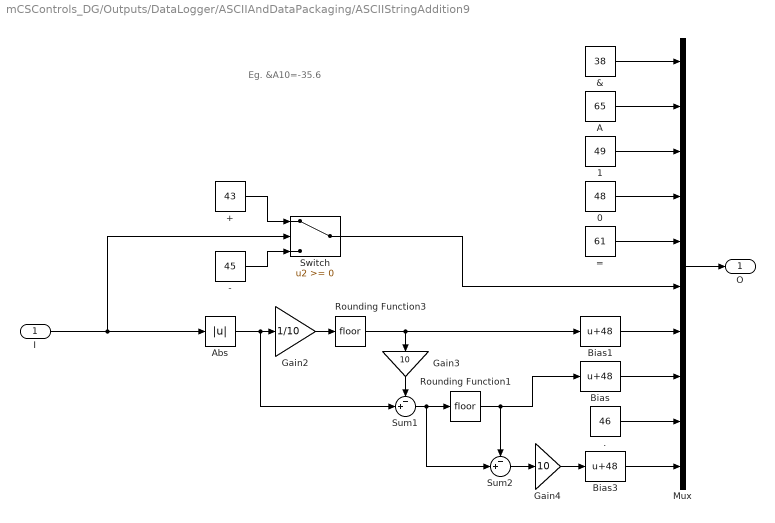
== system mCSControls_DG/Outputs/DataLogger/ASCIIAndDataPackaging/ASCIIStringAddition9 ==
  note: Eg. &A10=-35.6
  I : Inport
  & : Constant  Value=38
  + : Constant  Value=43
  - : Constant  Value=45
  . : Constant  Value=46
  0 : Constant  Value=48
  1 : Constant  Value=49
  = : Constant  Value=61
  A : Constant  Value=65
  Abs : Abs
  Bias : Bias  Bias=48
  Bias1 : Bias  Bias=48
  Bias3 : Bias  Bias=48
  Gain2 : Gain  Gain=1/10
  Gain3 : Gain  Gain=10
  Gain4 : Gain  Gain=10
  Mux : Mux  Inputs=10
  Rounding Function1 : Rounding
  Rounding Function3 : Rounding
  Sum1 : Sum  Inputs=-+|
  Sum2 : Sum  Inputs=-+|
  Switch : Switch
  O : Outport
  wires:
  ./1 -> Mux/9
  Bias/1 -> Mux/8
  Bias1/1 -> Mux/7
  Bias3/1 -> Mux/10
  Switch/1 -> Mux/6
  =/1 -> Mux/5
  0/1 -> Mux/4
  1/1 -> Mux/3
  A/1 -> Mux/2
  &/1 -> Mux/1
  I/1 -> Abs/1, Switch/2
  +/1 -> Switch/1
  -/1 -> Switch/3
  Abs/1 -> Gain2/1, Sum1/2
  Gain3/1 -> Sum1/1
  Rounding Function3/1 -> Bias1/1, Gain3/1
  Gain2/1 -> Rounding Function3/1
  Mux/1 -> O/1
  Sum1/1 -> Sum2/2, Rounding Function1/1
  Rounding Function1/1 -> Bias/1, Sum2/1
  Sum2/1 -> Gain4/1
  Gain4/1 -> Bias3/1

== system mCSControls_DG/Outputs/DataLogger/Debugging/ASCII Conversion ==
  I : Inport
  Bias : Bias  Bias=48
  Bias1 : Bias  Bias=48
  Bias2 : Bias  Bias=48
  Gain : Gain  Gain=1/100
  Gain1 : Gain  Gain=100
  Gain2 : Gain  Gain=1/10
  Gain3 : Gain  Gain=10
  Mux : Mux
  Rounding Function : Rounding
  Rounding Function3 : Rounding
  Space : Constant  Value=32
  Sum : Sum  Inputs=-+|
  Sum1 : Sum  Inputs=-+|
  O : Outport
  wires:
  Mux/1 -> O/1
  Space/1 -> Mux/4
  Bias/1 -> Mux/3
  Bias1/1 -> Mux/2
  Bias2/1 -> Mux/1
  Gain/1 -> Rounding Function/1
  I/1 -> Sum/2, Gain/1
  Gain1/1 -> Sum/1
  Rounding Function/1 -> Bias2/1, Gain1/1
  Sum/1 -> Sum1/2, Gain2/1
  Gain2/1 -> Rounding Function3/1
  Rounding Function3/1 -> Bias1/1, Gain3/1
  Gain3/1 -> Sum1/1
  Sum1/1 -> Bias/1

== system mCSControls_DG/Outputs/DataLogger/Debugging/ASCII Conversion1 ==
  I : Inport
  Bias : Bias  Bias=48
  Bias1 : Bias  Bias=48
  Bias2 : Bias  Bias=48
  Gain : Gain  Gain=1/100
  Gain1 : Gain  Gain=100
  Gain2 : Gain  Gain=1/10
  Gain3 : Gain  Gain=10
  Mux : Mux
  Rounding Function : Rounding
  Rounding Function3 : Rounding
  Space : Constant  Value=32
  Sum : Sum  Inputs=-+|
  Sum1 : Sum  Inputs=-+|
  O : Outport
  wires:
  Sum1/1 -> Bias/1
  Gain3/1 -> Sum1/1
  Rounding Function3/1 -> Gain3/1, Bias1/1
  Gain2/1 -> Rounding Function3/1
  Sum/1 -> Gain2/1, Sum1/2
  Rounding Function/1 -> Gain1/1, Bias2/1
  Gain1/1 -> Sum/1
  I/1 -> Gain/1, Sum/2
  Gain/1 -> Rounding Function/1
  Bias2/1 -> Mux/1
  Bias1/1 -> Mux/2
  Bias/1 -> Mux/3
  Space/1 -> Mux/4
  Mux/1 -> O/1

== system mCSControls_DG/Outputs/DataLogger/Debugging/ASCII Conversion10 ==
  I : Inport
  Bias : Bias  Bias=48
  Bias1 : Bias  Bias=48
  Bias2 : Bias  Bias=48
  Gain : Gain  Gain=1/100
  Gain1 : Gain  Gain=100
  Gain2 : Gain  Gain=1/10
  Gain3 : Gain  Gain=10
  Mux : Mux
  Rounding Function : Rounding
  Rounding Function3 : Rounding
  Space : Constant  Value=32
  Sum : Sum  Inputs=-+|
  Sum1 : Sum  Inputs=-+|
  O : Outport
  wires:
  Mux/1 -> O/1
  Space/1 -> Mux/4
  Bias/1 -> Mux/3
  Bias1/1 -> Mux/2
  Bias2/1 -> Mux/1
  Gain/1 -> Rounding Function/1
  I/1 -> Sum/2, Gain/1
  Gain1/1 -> Sum/1
  Rounding Function/1 -> Bias2/1, Gain1/1
  Sum/1 -> Sum1/2, Gain2/1
  Gain2/1 -> Rounding Function3/1
  Rounding Function3/1 -> Bias1/1, Gain3/1
  Gain3/1 -> Sum1/1
  Sum1/1 -> Bias/1

== system mCSControls_DG/Outputs/DataLogger/Debugging/ASCII Conversion11 ==
  I : Inport
  Bias : Bias  Bias=48
  Bias1 : Bias  Bias=48
  Bias2 : Bias  Bias=48
  Gain : Gain  Gain=1/100
  Gain1 : Gain  Gain=100
  Gain2 : Gain  Gain=1/10
  Gain3 : Gain  Gain=10
  Mux : Mux
  Rounding Function : Rounding
  Rounding Function3 : Rounding
  Space : Constant  Value=32
  Sum : Sum  Inputs=-+|
  Sum1 : Sum  Inputs=-+|
  O : Outport
  wires:
  Sum1/1 -> Bias/1
  Gain3/1 -> Sum1/1
  Rounding Function3/1 -> Gain3/1, Bias1/1
  Gain2/1 -> Rounding Function3/1
  Sum/1 -> Gain2/1, Sum1/2
  Rounding Function/1 -> Gain1/1, Bias2/1
  Gain1/1 -> Sum/1
  I/1 -> Gain/1, Sum/2
  Gain/1 -> Rounding Function/1
  Bias2/1 -> Mux/1
  Bias1/1 -> Mux/2
  Bias/1 -> Mux/3
  Space/1 -> Mux/4
  Mux/1 -> O/1

== system mCSControls_DG/Outputs/DataLogger/Debugging/ASCII Conversion12 ==
  I : Inport
  Bias : Bias  Bias=48
  Bias1 : Bias  Bias=48
  Bias2 : Bias  Bias=48
  Gain : Gain  Gain=1/100
  Gain1 : Gain  Gain=100
  Gain2 : Gain  Gain=1/10
  Gain3 : Gain  Gain=10
  Mux : Mux
  Rounding Function : Rounding
  Rounding Function3 : Rounding
  Space : Constant  Value=32
  Sum : Sum  Inputs=-+|
  Sum1 : Sum  Inputs=-+|
  O : Outport
  wires:
  Mux/1 -> O/1
  Space/1 -> Mux/4
  Bias/1 -> Mux/3
  Bias1/1 -> Mux/2
  Bias2/1 -> Mux/1
  Gain/1 -> Rounding Function/1
  I/1 -> Sum/2, Gain/1
  Gain1/1 -> Sum/1
  Rounding Function/1 -> Bias2/1, Gain1/1
  Sum/1 -> Sum1/2, Gain2/1
  Gain2/1 -> Rounding Function3/1
  Rounding Function3/1 -> Bias1/1, Gain3/1
  Gain3/1 -> Sum1/1
  Sum1/1 -> Bias/1

== system mCSControls_DG/Outputs/DataLogger/Debugging/ASCII Conversion13 ==
  I : Inport
  Bias : Bias  Bias=48
  Bias1 : Bias  Bias=48
  Bias2 : Bias  Bias=48
  Gain : Gain  Gain=1/100
  Gain1 : Gain  Gain=100
  Gain2 : Gain  Gain=1/10
  Gain3 : Gain  Gain=10
  Mux : Mux
  Rounding Function : Rounding
  Rounding Function3 : Rounding
  Space : Constant  Value=32
  Sum : Sum  Inputs=-+|
  Sum1 : Sum  Inputs=-+|
  O : Outport
  wires:
  Sum1/1 -> Bias/1
  Gain3/1 -> Sum1/1
  Rounding Function3/1 -> Gain3/1, Bias1/1
  Gain2/1 -> Rounding Function3/1
  Sum/1 -> Gain2/1, Sum1/2
  Rounding Function/1 -> Gain1/1, Bias2/1
  Gain1/1 -> Sum/1
  I/1 -> Gain/1, Sum/2
  Gain/1 -> Rounding Function/1
  Bias2/1 -> Mux/1
  Bias1/1 -> Mux/2
  Bias/1 -> Mux/3
  Space/1 -> Mux/4
  Mux/1 -> O/1

== system mCSControls_DG/Outputs/DataLogger/Debugging/ASCII Conversion14 ==
  I : Inport
  Bias : Bias  Bias=48
  Bias1 : Bias  Bias=48
  Bias2 : Bias  Bias=48
  Gain : Gain  Gain=1/100
  Gain1 : Gain  Gain=100
  Gain2 : Gain  Gain=1/10
  Gain3 : Gain  Gain=10
  Mux : Mux
  Rounding Function : Rounding
  Rounding Function3 : Rounding
  Space : Constant  Value=32
  Sum : Sum  Inputs=-+|
  Sum1 : Sum  Inputs=-+|
  O : Outport
  wires:
  Mux/1 -> O/1
  Space/1 -> Mux/4
  Bias/1 -> Mux/3
  Bias1/1 -> Mux/2
  Bias2/1 -> Mux/1
  Gain/1 -> Rounding Function/1
  I/1 -> Sum/2, Gain/1
  Gain1/1 -> Sum/1
  Rounding Function/1 -> Bias2/1, Gain1/1
  Sum/1 -> Sum1/2, Gain2/1
  Gain2/1 -> Rounding Function3/1
  Rounding Function3/1 -> Bias1/1, Gain3/1
  Gain3/1 -> Sum1/1
  Sum1/1 -> Bias/1

== system mCSControls_DG/Outputs/DataLogger/Debugging/ASCII Conversion15 ==
  I : Inport
  Bias : Bias  Bias=48
  Bias1 : Bias  Bias=48
  Bias2 : Bias  Bias=48
  Gain : Gain  Gain=1/100
  Gain1 : Gain  Gain=100
  Gain2 : Gain  Gain=1/10
  Gain3 : Gain  Gain=10
  Mux : Mux
  Rounding Function : Rounding
  Rounding Function3 : Rounding
  Space : Constant  Value=32
  Sum : Sum  Inputs=-+|
  Sum1 : Sum  Inputs=-+|
  O : Outport
  wires:
  Sum1/1 -> Bias/1
  Gain3/1 -> Sum1/1
  Rounding Function3/1 -> Gain3/1, Bias1/1
  Gain2/1 -> Rounding Function3/1
  Sum/1 -> Gain2/1, Sum1/2
  Rounding Function/1 -> Gain1/1, Bias2/1
  Gain1/1 -> Sum/1
  I/1 -> Gain/1, Sum/2
  Gain/1 -> Rounding Function/1
  Bias2/1 -> Mux/1
  Bias1/1 -> Mux/2
  Bias/1 -> Mux/3
  Space/1 -> Mux/4
  Mux/1 -> O/1

== system mCSControls_DG/Outputs/DataLogger/Debugging/ASCII Conversion16 ==
  I : Inport
  Bias : Bias  Bias=48
  Bias1 : Bias  Bias=48
  Bias2 : Bias  Bias=48
  Gain : Gain  Gain=1/100
  Gain1 : Gain  Gain=100
  Gain2 : Gain  Gain=1/10
  Gain3 : Gain  Gain=10
  Mux : Mux
  Rounding Function : Rounding
  Rounding Function3 : Rounding
  Space : Constant  Value=32
  Sum : Sum  Inputs=-+|
  Sum1 : Sum  Inputs=-+|
  O : Outport
  wires:
  Mux/1 -> O/1
  Space/1 -> Mux/4
  Bias/1 -> Mux/3
  Bias1/1 -> Mux/2
  Bias2/1 -> Mux/1
  Gain/1 -> Rounding Function/1
  I/1 -> Sum/2, Gain/1
  Gain1/1 -> Sum/1
  Rounding Function/1 -> Bias2/1, Gain1/1
  Sum/1 -> Sum1/2, Gain2/1
  Gain2/1 -> Rounding Function3/1
  Rounding Function3/1 -> Bias1/1, Gain3/1
  Gain3/1 -> Sum1/1
  Sum1/1 -> Bias/1

== system mCSControls_DG/Outputs/DataLogger/Debugging/ASCII Conversion17 ==
  I : Inport
  Bias : Bias  Bias=48
  Bias1 : Bias  Bias=48
  Bias2 : Bias  Bias=48
  Gain : Gain  Gain=1/100
  Gain1 : Gain  Gain=100
  Gain2 : Gain  Gain=1/10
  Gain3 : Gain  Gain=10
  Mux : Mux
  Rounding Function : Rounding
  Rounding Function3 : Rounding
  Space : Constant  Value=32
  Sum : Sum  Inputs=-+|
  Sum1 : Sum  Inputs=-+|
  O : Outport
  wires:
  Sum1/1 -> Bias/1
  Gain3/1 -> Sum1/1
  Rounding Function3/1 -> Gain3/1, Bias1/1
  Gain2/1 -> Rounding Function3/1
  Sum/1 -> Gain2/1, Sum1/2
  Rounding Function/1 -> Gain1/1, Bias2/1
  Gain1/1 -> Sum/1
  I/1 -> Gain/1, Sum/2
  Gain/1 -> Rounding Function/1
  Bias2/1 -> Mux/1
  Bias1/1 -> Mux/2
  Bias/1 -> Mux/3
  Space/1 -> Mux/4
  Mux/1 -> O/1

== system mCSControls_DG/Outputs/DataLogger/Debugging/ASCII Conversion18 ==
  I : Inport
  Bias : Bias  Bias=48
  Bias1 : Bias  Bias=48
  Bias2 : Bias  Bias=48
  Gain : Gain  Gain=1/100
  Gain1 : Gain  Gain=100
  Gain2 : Gain  Gain=1/10
  Gain3 : Gain  Gain=10
  Mux : Mux
  Rounding Function : Rounding
  Rounding Function3 : Rounding
  Space : Constant  Value=32
  Sum : Sum  Inputs=-+|
  Sum1 : Sum  Inputs=-+|
  O : Outport
  wires:
  Mux/1 -> O/1
  Space/1 -> Mux/4
  Bias/1 -> Mux/3
  Bias1/1 -> Mux/2
  Bias2/1 -> Mux/1
  Gain/1 -> Rounding Function/1
  I/1 -> Sum/2, Gain/1
  Gain1/1 -> Sum/1
  Rounding Function/1 -> Bias2/1, Gain1/1
  Sum/1 -> Sum1/2, Gain2/1
  Gain2/1 -> Rounding Function3/1
  Rounding Function3/1 -> Bias1/1, Gain3/1
  Gain3/1 -> Sum1/1
  Sum1/1 -> Bias/1

== system mCSControls_DG/Outputs/DataLogger/Debugging/ASCII Conversion19 ==
  I : Inport
  Bias : Bias  Bias=48
  Bias1 : Bias  Bias=48
  Bias2 : Bias  Bias=48
  Gain : Gain  Gain=1/100
  Gain1 : Gain  Gain=100
  Gain2 : Gain  Gain=1/10
  Gain3 : Gain  Gain=10
  Mux : Mux
  Rounding Function : Rounding
  Rounding Function3 : Rounding
  Space : Constant  Value=32
  Sum : Sum  Inputs=-+|
  Sum1 : Sum  Inputs=-+|
  O : Outport
  wires:
  Sum1/1 -> Bias/1
  Gain3/1 -> Sum1/1
  Rounding Function3/1 -> Gain3/1, Bias1/1
  Gain2/1 -> Rounding Function3/1
  Sum/1 -> Gain2/1, Sum1/2
  Rounding Function/1 -> Gain1/1, Bias2/1
  Gain1/1 -> Sum/1
  I/1 -> Gain/1, Sum/2
  Gain/1 -> Rounding Function/1
  Bias2/1 -> Mux/1
  Bias1/1 -> Mux/2
  Bias/1 -> Mux/3
  Space/1 -> Mux/4
  Mux/1 -> O/1

== system mCSControls_DG/Outputs/DataLogger/Debugging/ASCII Conversion2 ==
  I : Inport
  Bias : Bias  Bias=48
  Bias1 : Bias  Bias=48
  Bias2 : Bias  Bias=48
  Gain : Gain  Gain=1/100
  Gain1 : Gain  Gain=100
  Gain2 : Gain  Gain=1/10
  Gain3 : Gain  Gain=10
  Mux : Mux
  Rounding Function : Rounding
  Rounding Function3 : Rounding
  Space : Constant  Value=32
  Sum : Sum  Inputs=-+|
  Sum1 : Sum  Inputs=-+|
  O : Outport
  wires:
  Mux/1 -> O/1
  Space/1 -> Mux/4
  Bias/1 -> Mux/3
  Bias1/1 -> Mux/2
  Bias2/1 -> Mux/1
  Gain/1 -> Rounding Function/1
  I/1 -> Sum/2, Gain/1
  Gain1/1 -> Sum/1
  Rounding Function/1 -> Bias2/1, Gain1/1
  Sum/1 -> Sum1/2, Gain2/1
  Gain2/1 -> Rounding Function3/1
  Rounding Function3/1 -> Bias1/1, Gain3/1
  Gain3/1 -> Sum1/1
  Sum1/1 -> Bias/1

== system mCSControls_DG/Outputs/DataLogger/Debugging/ASCII Conversion3 ==
  I : Inport
  Bias : Bias  Bias=48
  Bias1 : Bias  Bias=48
  Bias2 : Bias  Bias=48
  Gain : Gain  Gain=1/100
  Gain1 : Gain  Gain=100
  Gain2 : Gain  Gain=1/10
  Gain3 : Gain  Gain=10
  Mux : Mux
  Rounding Function : Rounding
  Rounding Function3 : Rounding
  Space : Constant  Value=32
  Sum : Sum  Inputs=-+|
  Sum1 : Sum  Inputs=-+|
  O : Outport
  wires:
  Sum1/1 -> Bias/1
  Gain3/1 -> Sum1/1
  Rounding Function3/1 -> Gain3/1, Bias1/1
  Gain2/1 -> Rounding Function3/1
  Sum/1 -> Gain2/1, Sum1/2
  Rounding Function/1 -> Gain1/1, Bias2/1
  Gain1/1 -> Sum/1
  I/1 -> Gain/1, Sum/2
  Gain/1 -> Rounding Function/1
  Bias2/1 -> Mux/1
  Bias1/1 -> Mux/2
  Bias/1 -> Mux/3
  Space/1 -> Mux/4
  Mux/1 -> O/1

== system mCSControls_DG/Outputs/DataLogger/Debugging/ASCII Conversion4 ==
  I : Inport
  Bias : Bias  Bias=48
  Bias1 : Bias  Bias=48
  Bias2 : Bias  Bias=48
  Gain : Gain  Gain=1/100
  Gain1 : Gain  Gain=100
  Gain2 : Gain  Gain=1/10
  Gain3 : Gain  Gain=10
  Mux : Mux
  Rounding Function : Rounding
  Rounding Function3 : Rounding
  Space : Constant  Value=32
  Sum : Sum  Inputs=-+|
  Sum1 : Sum  Inputs=-+|
  O : Outport
  wires:
  Mux/1 -> O/1
  Space/1 -> Mux/4
  Bias/1 -> Mux/3
  Bias1/1 -> Mux/2
  Bias2/1 -> Mux/1
  Gain/1 -> Rounding Function/1
  I/1 -> Sum/2, Gain/1
  Gain1/1 -> Sum/1
  Rounding Function/1 -> Bias2/1, Gain1/1
  Sum/1 -> Sum1/2, Gain2/1
  Gain2/1 -> Rounding Function3/1
  Rounding Function3/1 -> Bias1/1, Gain3/1
  Gain3/1 -> Sum1/1
  Sum1/1 -> Bias/1

== system mCSControls_DG/Outputs/DataLogger/Debugging/ASCII Conversion5 ==
  I : Inport
  Bias : Bias  Bias=48
  Bias1 : Bias  Bias=48
  Bias2 : Bias  Bias=48
  Gain : Gain  Gain=1/100
  Gain1 : Gain  Gain=100
  Gain2 : Gain  Gain=1/10
  Gain3 : Gain  Gain=10
  Mux : Mux
  Rounding Function : Rounding
  Rounding Function3 : Rounding
  Space : Constant  Value=32
  Sum : Sum  Inputs=-+|
  Sum1 : Sum  Inputs=-+|
  O : Outport
  wires:
  Sum1/1 -> Bias/1
  Gain3/1 -> Sum1/1
  Rounding Function3/1 -> Gain3/1, Bias1/1
  Gain2/1 -> Rounding Function3/1
  Sum/1 -> Gain2/1, Sum1/2
  Rounding Function/1 -> Gain1/1, Bias2/1
  Gain1/1 -> Sum/1
  I/1 -> Gain/1, Sum/2
  Gain/1 -> Rounding Function/1
  Bias2/1 -> Mux/1
  Bias1/1 -> Mux/2
  Bias/1 -> Mux/3
  Space/1 -> Mux/4
  Mux/1 -> O/1

== system mCSControls_DG/Outputs/DataLogger/Debugging/ASCII Conversion6 ==
  I : Inport
  Bias : Bias  Bias=48
  Bias1 : Bias  Bias=48
  Bias2 : Bias  Bias=48
  Gain : Gain  Gain=1/100
  Gain1 : Gain  Gain=100
  Gain2 : Gain  Gain=1/10
  Gain3 : Gain  Gain=10
  Mux : Mux
  Rounding Function : Rounding
  Rounding Function3 : Rounding
  Space : Constant  Value=32
  Sum : Sum  Inputs=-+|
  Sum1 : Sum  Inputs=-+|
  O : Outport
  wires:
  Mux/1 -> O/1
  Space/1 -> Mux/4
  Bias/1 -> Mux/3
  Bias1/1 -> Mux/2
  Bias2/1 -> Mux/1
  Gain/1 -> Rounding Function/1
  I/1 -> Sum/2, Gain/1
  Gain1/1 -> Sum/1
  Rounding Function/1 -> Bias2/1, Gain1/1
  Sum/1 -> Sum1/2, Gain2/1
  Gain2/1 -> Rounding Function3/1
  Rounding Function3/1 -> Bias1/1, Gain3/1
  Gain3/1 -> Sum1/1
  Sum1/1 -> Bias/1

== system mCSControls_DG/Outputs/DataLogger/Debugging/ASCII Conversion7 ==
  I : Inport
  Bias : Bias  Bias=48
  Bias1 : Bias  Bias=48
  Bias2 : Bias  Bias=48
  Gain : Gain  Gain=1/100
  Gain1 : Gain  Gain=100
  Gain2 : Gain  Gain=1/10
  Gain3 : Gain  Gain=10
  Mux : Mux
  Rounding Function : Rounding
  Rounding Function3 : Rounding
  Space : Constant  Value=32
  Sum : Sum  Inputs=-+|
  Sum1 : Sum  Inputs=-+|
  O : Outport
  wires:
  Sum1/1 -> Bias/1
  Gain3/1 -> Sum1/1
  Rounding Function3/1 -> Gain3/1, Bias1/1
  Gain2/1 -> Rounding Function3/1
  Sum/1 -> Gain2/1, Sum1/2
  Rounding Function/1 -> Gain1/1, Bias2/1
  Gain1/1 -> Sum/1
  I/1 -> Gain/1, Sum/2
  Gain/1 -> Rounding Function/1
  Bias2/1 -> Mux/1
  Bias1/1 -> Mux/2
  Bias/1 -> Mux/3
  Space/1 -> Mux/4
  Mux/1 -> O/1

== system mCSControls_DG/Outputs/DataLogger/Debugging/ASCII Conversion8 ==
  I : Inport
  Bias : Bias  Bias=48
  Bias1 : Bias  Bias=48
  Bias2 : Bias  Bias=48
  Gain : Gain  Gain=1/100
  Gain1 : Gain  Gain=100
  Gain2 : Gain  Gain=1/10
  Gain3 : Gain  Gain=10
  Mux : Mux
  Rounding Function : Rounding
  Rounding Function3 : Rounding
  Space : Constant  Value=32
  Sum : Sum  Inputs=-+|
  Sum1 : Sum  Inputs=-+|
  O : Outport
  wires:
  Mux/1 -> O/1
  Space/1 -> Mux/4
  Bias/1 -> Mux/3
  Bias1/1 -> Mux/2
  Bias2/1 -> Mux/1
  Gain/1 -> Rounding Function/1
  I/1 -> Sum/2, Gain/1
  Gain1/1 -> Sum/1
  Rounding Function/1 -> Bias2/1, Gain1/1
  Sum/1 -> Sum1/2, Gain2/1
  Gain2/1 -> Rounding Function3/1
  Rounding Function3/1 -> Bias1/1, Gain3/1
  Gain3/1 -> Sum1/1
  Sum1/1 -> Bias/1

== system mCSControls_DG/Outputs/DataLogger/Debugging/ASCII Conversion9 ==
  I : Inport
  Bias : Bias  Bias=48
  Bias1 : Bias  Bias=48
  Bias2 : Bias  Bias=48
  Gain : Gain  Gain=1/100
  Gain1 : Gain  Gain=100
  Gain2 : Gain  Gain=1/10
  Gain3 : Gain  Gain=10
  Mux : Mux
  Rounding Function : Rounding
  Rounding Function3 : Rounding
  Space : Constant  Value=32
  Sum : Sum  Inputs=-+|
  Sum1 : Sum  Inputs=-+|
  O : Outport
  wires:
  Sum1/1 -> Bias/1
  Gain3/1 -> Sum1/1
  Rounding Function3/1 -> Gain3/1, Bias1/1
  Gain2/1 -> Rounding Function3/1
  Sum/1 -> Gain2/1, Sum1/2
  Rounding Function/1 -> Gain1/1, Bias2/1
  Gain1/1 -> Sum/1
  I/1 -> Gain/1, Sum/2
  Gain/1 -> Rounding Function/1
  Bias2/1 -> Mux/1
  Bias1/1 -> Mux/2
  Bias/1 -> Mux/3
  Space/1 -> Mux/4
  Mux/1 -> O/1

== system mCSControls_DG/Outputs/LCD/Transmit/LEDOnPanelBox ==
  P : Inport
  TH1Achieved : Inport  Port=2
  Compare To Zero : simulink/Logic and Bit Operations/Compare To Zero  relop=<=  OutDataTypeStr=uint8
  Compare To Zero1 : simulink/Logic and Bit Operations/Compare To Zero  relop=>  OutDataTypeStr=uint8
  Compare To Zero2 : simulink/Logic and Bit Operations/Compare To Zero  relop=<=  OutDataTypeStr=uint8
  Green : c2833xlib/Digital Output  GPIO_Number=GPIO16~GPIO23  GPIO_Bit0=off  GPIO_BIT0_Toggle=off  GPIO_Bit1=on  GPIO_BIT1_Toggle=off  GPIO_Bit2=off  GPIO_BIT2_Toggle=off  GPIO_Bit3=off  GPIO_BIT3_Toggle=off  GPIO_Bit4=off  GPIO_BIT4_Toggle=off  GPIO_Bit5=off  GPIO_BIT5_Toggle=off  GPIO_Bit6=off  GPIO_BIT6_Toggle=off  GPIO_Bit7=off  GPIO_BIT7_Toggle=off
  Orange : c2833xlib/Digital Output  GPIO_Number=GPIO16~GPIO23  GPIO_Bit0=off  GPIO_BIT0_Toggle=off  GPIO_Bit1=off  GPIO_BIT1_Toggle=off  GPIO_Bit2=off  GPIO_BIT2_Toggle=off  GPIO_Bit3=on  GPIO_BIT3_Toggle=off  GPIO_Bit4=off  GPIO_BIT4_Toggle=off  GPIO_Bit5=off  GPIO_BIT5_Toggle=off  GPIO_Bit6=off  GPIO_BIT6_Toggle=off  GPIO_Bit7=off  GPIO_BIT7_Toggle=off
  Product : Product  RndMeth=Zero
  Product1 : Product  RndMeth=Zero
  Red : c2833xlib/Digital Output  GPIO_Number=GPIO16~GPIO23  GPIO_Bit0=off  GPIO_BIT0_Toggle=off  GPIO_Bit1=off  GPIO_BIT1_Toggle=off  GPIO_Bit2=off  GPIO_BIT2_Toggle=off  GPIO_Bit3=off  GPIO_BIT3_Toggle=off  GPIO_Bit4=off  GPIO_BIT4_Toggle=off  GPIO_Bit5=on  GPIO_BIT5_Toggle=off  GPIO_Bit6=off  GPIO_BIT6_Toggle=off  GPIO_Bit7=off  GPIO_BIT7_Toggle=off
  wires:
  Compare To Zero/1 -> Red/1  "Red"
  Compare To Zero1/1 -> Product1/1, Product/1
  P/1 -> Compare To Zero1/1, Compare To Zero/1
  Product/1 -> Orange/1
  Product1/1 -> Green/1
  TH1Achieved/1 -> Product1/2, Compare To Zero2/1
  Compare To Zero2/1 -> Product/2

== system mCSControls_DG/Outputs/LCD/Transmit/SetpointAchieved ==
  TH1 : Inport
  B : Inport  Port=2
  Bias : Bias  Bias=1
  Data Type Conversion : DataTypeConversion
  Relational Operator : RelationalOperator  Operator=<=  OutDataTypeStr=boolean
  Selector : Selector  IndexOptions=Index vector (port)  Indices=[1 3]  OutputSizes=1
  TempSetPoints : Constant  Value=T
  LED : Outport
  wires:
  TempSetPoints/1 -> Selector/1
  B/1 -> Selector/2
  Relational Operator/1 -> Data Type Conversion/1
  Selector/1 -> Bias/1
  Data Type Conversion/1 -> LED/1
  TH1/1 -> Relational Operator/1
  Bias/1 -> Relational Operator/2

== system mCSControls_DG/Inputs/DriveParams/DriveParamReceive/Rx/FAULTSRx ==
  SCIBRx : Inport
  Enable : EnablePort
  CRC-16L : Terminator
  CRC-16U : Terminator
  Data Type Conversion : DataTypeConversion  OutDataTypeStr=double
  Data Type Conversion1 : DataTypeConversion  OutDataTypeStr=uint16
  DataQuantity : Terminator
  Demux : Demux  Outputs=15
  FunctionCount : Terminator
  Gain : Gain  Gain=256  OutDataTypeStr=uint16
  Loopback{1..8} (8 alike) : Terminator
  SlaveAddress : Terminator
  Sum : Sum  Inputs=|++
  D : Outport
  wires:
  Demux/13 -> Sum/2
  Demux/12 -> Data Type Conversion1/1
  Demux/14 -> CRC-16U/1
  Demux/15 -> CRC-16L/1
  Demux/11 -> DataQuantity/1
  Demux/10 -> FunctionCount/1
  Demux/9 -> SlaveAddress/1
  Demux/8 -> Loopback8/1
  Demux/7 -> Loopback7/1
  Demux/6 -> Loopback6/1
  Demux/5 -> Loopback5/1
  Demux/4 -> Loopback4/1
  Demux/3 -> Loopback3/1
  Demux/2 -> Loopback2/1
  Demux/1 -> Loopback1/1
  Gain/1 -> Sum/1
  SCIBRx/1 -> Demux/1
  Data Type Conversion1/1 -> Gain/1
  Data Type Conversion/1 -> D/1
  Sum/1 -> Data Type Conversion/1  "PFreq"

== system mCSControls_DG/Inputs/DriveParams/DriveParamReceive/Rx/OPCurrRx ==
  SCIBRx : Inport
  Enable : EnablePort
  CRC-16L : Terminator
  CRC-16U : Terminator
  Data Type Conversion : DataTypeConversion  OutDataTypeStr=double
  Data Type Conversion1 : DataTypeConversion  OutDataTypeStr=uint16
  DataQuantity : Terminator
  Demux : Demux  Outputs=15
  FunctionCount : Terminator
  Gain : Gain  Gain=256  OutDataTypeStr=uint16
  Gain1 : Gain  Gain=0.1
  Loopback{1..8} (8 alike) : Terminator
  SlaveAddress : Terminator
  Sum : Sum  Inputs=|++
  D : Outport
  wires:
  Data Type Conversion1/1 -> Gain/1
  SCIBRx/1 -> Demux/1
  Gain/1 -> Sum/1
  Demux/1 -> Loopback1/1
  Demux/2 -> Loopback2/1
  Demux/3 -> Loopback3/1
  Demux/4 -> Loopback4/1
  Demux/5 -> Loopback5/1
  Demux/6 -> Loopback6/1
  Demux/7 -> Loopback7/1
  Demux/8 -> Loopback8/1
  Demux/9 -> SlaveAddress/1
  Demux/10 -> FunctionCount/1
  Demux/11 -> DataQuantity/1
  Demux/15 -> CRC-16L/1
  Demux/14 -> CRC-16U/1
  Demux/12 -> Data Type Conversion1/1
  Demux/13 -> Sum/2
  Data Type Conversion/1 -> Gain1/1
  Sum/1 -> Data Type Conversion/1  "PFreq"
  Gain1/1 -> D/1
